simulink model "Gate"  (R2018a)
settings: Solver=VariableStepAuto  StartTime=0.0  StopTime=10.0  RelTol=1e-3
settings Model: Creator=Sadat Zubin Shah  LastModifiedBy=Sadat Zubin Shah

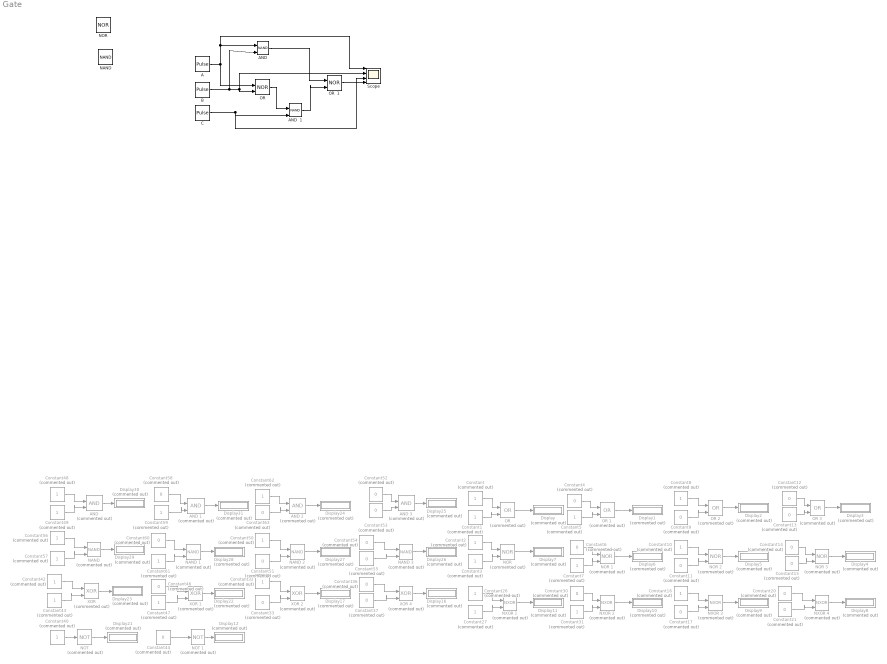
== system Gate ==
  A : DiscretePulseGenerator  PulseType=Time based  Period=10  PulseWidth=50
  AND {,1..3} (4 alike) : Logic  Commented=on  IconShape=distinctive  AllPortsSameDT=off  OutDataTypeStr=boolean
  "AND  " : Logic  Operator=NAND  IconShape=distinctive  AllPortsSameDT=off  OutDataTypeStr=boolean
  AND  1 : Logic  Operator=NAND  IconShape=distinctive  AllPortsSameDT=off  OutDataTypeStr=boolean
  B : DiscretePulseGenerator  PulseType=Time based  Period=5  PulseWidth=50
  C : DiscretePulseGenerator  PulseType=Time based  Period=2.5  PulseWidth=50
  Constant{,1..3,5,7..8,10,16,26..27,31..32,40,42..43,47..50,56..57,59,61..62} (25 alike) : Constant  Commented=on
  Constant{4,6,9,11..15,17,20..21,30,33,36..37,44,46,51..55,58,60,63} (25 alike) : Constant  Commented=on  Value=0
  Display{,1..12,16..17,21..31} (26 alike) : Display  Commented=on
  NAND : Logic  Operator=NAND  IconShape=distinctive  AllPortsSameDT=off  OutDataTypeStr=boolean
  NAND {,1..3} (4 alike) : Logic  Commented=on  Operator=NAND  IconShape=distinctive  AllPortsSameDT=off  OutDataTypeStr=boolean
  NOR : Logic  Operator=NOR  IconShape=distinctive  AllPortsSameDT=off  OutDataTypeStr=boolean
  NOR {,1..3} (4 alike) : Logic  Commented=on  Operator=NOR  IconShape=distinctive  AllPortsSameDT=off  OutDataTypeStr=boolean
  "NOT " : Logic  Commented=on  Operator=NOT  IconShape=distinctive  AllPortsSameDT=off  OutDataTypeStr=boolean
  NOT 1 : Logic  Commented=on  Operator=NOT  IconShape=distinctive  AllPortsSameDT=off  OutDataTypeStr=boolean
  NXOR {1..4} (4 alike) : Logic  Commented=on  Operator=NXOR  IconShape=distinctive  AllPortsSameDT=off  OutDataTypeStr=boolean
  OR {,1..3} (4 alike) : Logic  Commented=on  Operator=OR  IconShape=distinctive  AllPortsSameDT=off  OutDataTypeStr=boolean
  "OR  " : Logic  Operator=NOR  IconShape=distinctive  AllPortsSameDT=off  OutDataTypeStr=boolean
  OR  1 : Logic  Operator=NOR  IconShape=distinctive  AllPortsSameDT=off  OutDataTypeStr=boolean
  Scope : Scope  NumInputPorts=4
  XOR {,1..2,4} (4 alike) : Logic  Commented=on  Operator=XOR  IconShape=distinctive  AllPortsSameDT=off  OutDataTypeStr=boolean
  wires:
  OR 3/1 -> Display3/1
  NOR 1/1 -> Display6/1
  "NOR "/1 -> Display7/1
  "OR "/1 -> Display/1
  OR 1/1 -> Display1/1
  OR 2/1 -> Display2/1
  NOR 3/1 -> Display4/1
  NOR 2/1 -> Display5/1
  Constant/1 -> "OR "/1
  Constant1/1 -> "OR "/2
  Constant3/1 -> "NOR "/2
  Constant2/1 -> "NOR "/1
  Constant4/1 -> OR 1/1
  Constant5/1 -> OR 1/2
  Constant7/1 -> NOR 1/2
  Constant6/1 -> NOR 1/1
  Constant10/1 -> NOR 2/1
  Constant12/1 -> OR 3/1
  Constant13/1 -> OR 3/2
  Constant15/1 -> NOR 3/2
  Constant14/1 -> NOR 3/1
  Constant11/1 -> NOR 2/2
  Constant8/1 -> OR 2/1
  Constant62/1 -> AND 2/1
  Constant51/1 -> NAND 2/2
  Constant54/1 -> NAND 3/1
  Constant55/1 -> NAND 3/2
  Constant53/1 -> AND 3/2
  Constant52/1 -> AND 3/1
  Constant50/1 -> NAND 2/1
  Constant63/1 -> AND 2/2
  Constant60/1 -> NAND 1/1
  Constant61/1 -> NAND 1/2
  Constant59/1 -> AND 1/2
  Constant56/1 -> "NAND "/1
  Constant57/1 -> "NAND "/2
  Constant49/1 -> "AND "/2
  Constant48/1 -> "AND "/1
  NAND 2/1 -> Display27/1
  NAND 3/1 -> Display26/1
  AND 2/1 -> Display24/1
  AND 1/1 -> Display31/1
  "AND "/1 -> Display30/1
  "NAND "/1 -> Display29/1
  NAND 1/1 -> Display28/1
  AND 3/1 -> Display25/1
  XOR 1/1 -> Display22/1
  "XOR "/1 -> Display23/1
  XOR 4/1 -> Display16/1
  XOR 2/1 -> Display17/1
  Constant43/1 -> "XOR "/2
  Constant42/1 -> "XOR "/1
  Constant47/1 -> XOR 1/2
  Constant46/1 -> XOR 1/1
  Constant32/1 -> XOR 2/1
  Constant36/1 -> XOR 4/1
  Constant33/1 -> XOR 2/2
  Constant17/1 -> NXOR 3/2
  Constant20/1 -> NXOR 4/1
  Constant21/1 -> NXOR 4/2
  Constant16/1 -> NXOR 3/1
  Constant30/1 -> NXOR 2/1
  Constant31/1 -> NXOR 2/2
  Constant26/1 -> NXOR 1/1
  Constant27/1 -> NXOR 1/2
  NXOR 3/1 -> Display9/1
  NXOR 4/1 -> Display8/1
  NXOR 1/1 -> Display11/1
  NXOR 2/1 -> Display10/1
  Constant44/1 -> NOT 1/1
  Constant40/1 -> "NOT "/1
  "NOT "/1 -> Display21/1
  Constant58/1 -> AND 1/1
  Constant9/1 -> OR 2/2
  Constant37/1 -> XOR 4/2
  NOT 1/1 -> Display12/1
  A/1 -> "OR  "/1, Scope/1, "AND  "/1
  B/1 -> Scope/2, "OR  "/2, "AND  "/2
  C/1 -> Scope/3, AND  1/2
  "OR  "/1 -> AND  1/1
  AND  1/1 -> OR  1/2
  "AND  "/1 -> OR  1/1
  OR  1/1 -> Scope/4
